simulink model "gnc_rob_udp_sendrecieve_test"  (R2024b)
settings: Solver=VariableStepAuto  StartTime=0.0  StopTime=inf  FixedStep=0.05  RelTol=1e-3
libraries: nvidiaSharedBlocks x2
settings Model: Creator=SPOT  LastModifiedBy=SPOT

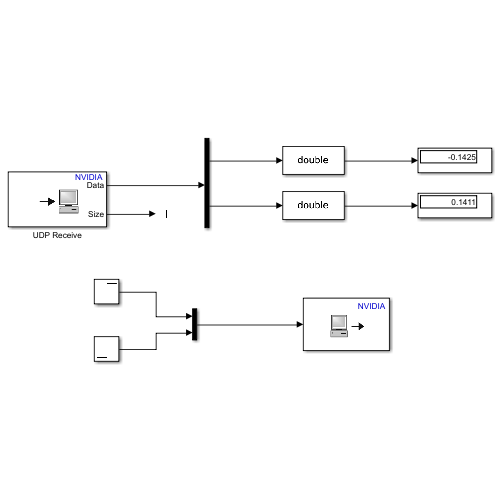
[thumbnail: Simulink's stored preview of the top-level diagram]
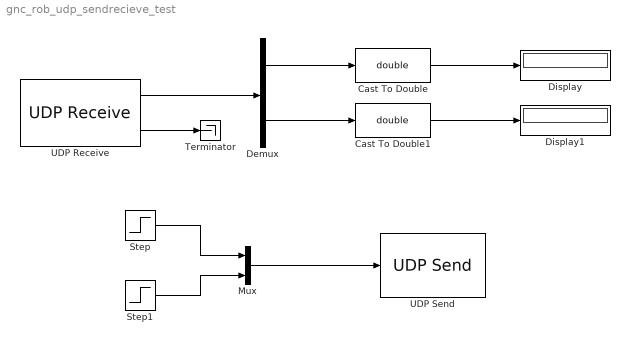
== system gnc_rob_udp_sendrecieve_test ==
  Cast To Double : DataTypeConversion  OutDataTypeStr=double  SaturateOnIntegerOverflow=off  RndMeth=Floor
  Cast To Double1 : DataTypeConversion  OutDataTypeStr=double  SaturateOnIntegerOverflow=off  RndMeth=Floor
  Demux : Demux  Outputs=2
  Display : Display
  Display1 : Display
  Mux : Mux  Inputs=2
  Step : Step  Time=10  SampleTime=0
  Step1 : Step  Time=100  SampleTime=0
  Terminator : Terminator
  UDP Receive : nvidiaSharedBlocks/UDP Receive  localURL='0.0.0.0'  localPort=13761  remoteURL='0.0.0.0'  remotePort=-1  recvBufferSize=8192  signalDatatype=single  dims=2  isVarSize=off  showBlockingTime=off  blockingTime=0  sampletime=baseRate  blockPlatform=NVIDIA
      settings: LibrarySourceBlock=nvidiaNetworklib/UDP Receive
  UDP Send : nvidiaSharedBlocks/UDP Send  remoteURL='192.168.1.30'  remotePort=10293  localURL='0.0.0.0'  localPortSource=Automatically determine  localPort=-1  sampletime=-1  blockPlatform=NVIDIA  separateLengthPort=0
      settings: LibrarySourceBlock=nvidiaNetworklib/UDP Send
  wires:
  UDP Receive/2 -> Terminator/1
  Cast To Double/1 -> Display/1
  UDP Receive/1 -> Demux/1
  Demux/1 -> Cast To Double/1
  Demux/2 -> Cast To Double1/1
  Cast To Double1/1 -> Display1/1
  Step/1 -> Mux/1
  Mux/1 -> UDP Send/1
  Step1/1 -> Mux/2
